simulink model "AAIR"  (R2020a)
settings: Solver=FixedStepAuto  StartTime=0.0  StopTime=60.0  FixedStep=1e-3  RelTol=1e-3  EnableMultiTasking=on
undefined symbols (not defined in the file): D0, D10, D11, D12, D13, D2, D4, D5, D6, D7, D8, D9, PTA0, PTA2, PTB23, PTB9, PTC16, PTC2, PTC3, PTC4, PTD0, PTD1, PTD2, PTD3
libraries: frdmk64flib x13, dspstat3 x1
settings Model: ExtModeTrigDuration=5  Creator=raymo  LastModifiedBy=raymo
settings OptimizationCC: EnhancedBackFolding=on  PassReuseOutputArgsAs=Individual arguments  ZeroExternalMemoryAtStartup=off  ZeroInternalMemoryAtStartup=off  MaxStackSize=64  OptimizeBlockOrder=speed  DifferentSizesBufferReuse=on  OptimizationCustomize=off  EfficientTunableParamExpr=on
settings DebuggingCC: ParameterTunabilityLossMsg=error
settings HardwareCC: ProdBitPerPointer=32  ProdBitPerSizeT=32  ProdBitPerPtrDiffT=32  ProdLargestAtomicInteger=Long  ProdLargestAtomicFloat=Double  ProdWordSize=32  ProdHWDeviceType=ARM Compatible->ARM Cortex
settings SFSimCC: MATLABDynamicMemAlloc=off
settings RTWCC: SystemTargetFile=ert.tlc  HardwareBoard=NXP FRDM-K64F  TemplateMakefile=ert_default_tmf  Toolchain=GNU Tools for ARM Embedded Processors
settings CodeAppCC: ForceParamTrailComments=on  IgnoreCustomStorageClasses=off  OperatorAnnotations=on  SimulinkDataObjDesc=on  SFDataObjDesc=on  InsertBlockDesc=on

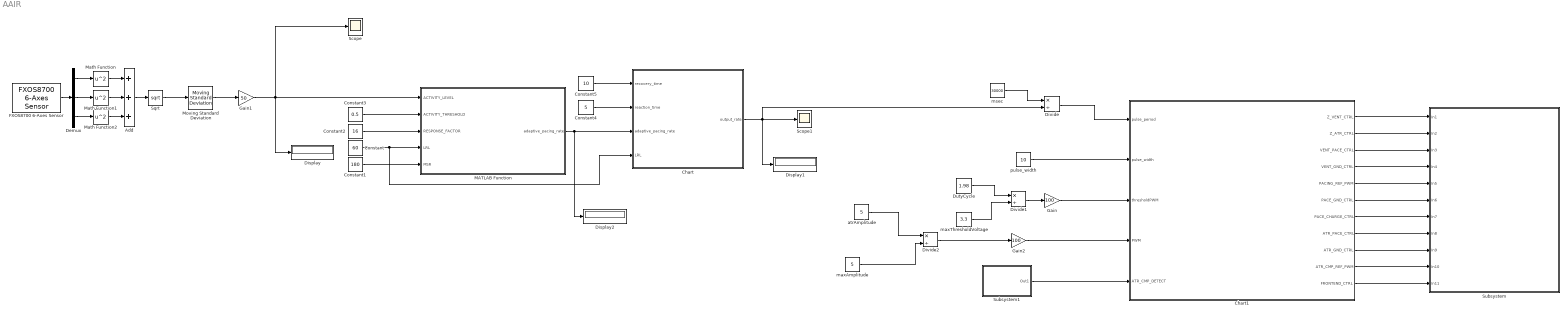
== system AAIR ==
  Add : Sum  Inputs=+++
  Chart : Stateflow chart  TreatAsAtomicUnit=on
  Chart1 : Stateflow chart  TreatAsAtomicUnit=on
  Constant : Constant  Value=60
  Constant1 : Constant  Value=180
  Constant2 : Constant  Value=16
  Constant3 : Constant  Value=0.5
  Constant4 : Constant  Value=5
  Constant5 : Constant  Value=10
  Demux : Demux  Outputs=3
  Display : Display
  Display1 : Display
  Display2 : Display
  Divide : Product  Inputs=*/
  Divide1 : Product  Inputs=*/
  Divide2 : Product  Inputs=*/
  DutyCycle : Constant  Value=1.98
  FXOS8700 6-Axes Sensor : frdmk64flib/FXOS8700 6-Axes Sensor  Activesensor=Accelerometer only  ODR=800Hz  HybridODR=400Hz  Accelfullrange=-4g to +4g  SampleTime=-1
  Gain : Gain  Gain=100
  Gain1 : Gain  Gain=50
  Gain2 : Gain  Gain=100
  MATLAB Function : MATLAB Function  TreatAsAtomicUnit=on
  Math Function : Math  Operator=square  SaturateOnIntegerOverflow=on
  Math Function1 : Math  Operator=square  SaturateOnIntegerOverflow=on
  Math Function2 : Math  Operator=square  SaturateOnIntegerOverflow=on
  Moving Standard Deviation : dspstat3/Moving Standard Deviation  Method=Sliding window  ForgettingFactorPort=off  SpecifyWindowLength=on  WindowLength=4  ForgettingFactor=0.9  SimulateUsing=Code generation
      settings: SourceProductBaseCode=DS
  Scope : Scope
  Scope1 : Scope
  Sqrt : Sqrt  SaturateOnIntegerOverflow=on
  Subsystem : Subsystem
  Subsystem1 : Subsystem
  atrAmplitude : Constant  Value=5
  maxAmplitude : Constant  Value=5
  maxThresholdVoltage : Constant  Value=3.3
  msec : Constant  Value=30000
  pulse_width : Constant  Value=10
  wires:
  Math Function2/1 -> Add/3
  Demux/3 -> Math Function2/1
  Constant2/1 -> MATLAB Function/3(RESPONSE_FACTOR)
  Constant/1 -> Chart/4(LRL), MATLAB Function/4(LRL)
  MATLAB Function/1(adaptive_pacing_rate) -> Chart/3(adaptive_pacing_rate), Display2/1
  Demux/1 -> Math Function/1
  Demux/2 -> Math Function1/1
  Math Function/1 -> Add/1
  Constant5/1 -> Chart/1(recovery_time)
  Add/1 -> Sqrt/1
  Constant4/1 -> Chart/2(reaction_time)
  Math Function1/1 -> Add/2
  Constant1/1 -> MATLAB Function/5(MSR)
  Sqrt/1 -> Moving Standard Deviation/1
  Gain1/1 -> Scope/1, Display/1, MATLAB Function/1(ACTIVITY_LEVEL)
  Constant3/1 -> MATLAB Function/2(ACTIVITY_THRESHOLD)
  FXOS8700 6-Axes Sensor/1 -> Demux/1
  Moving Standard Deviation/1 -> Gain1/1
  DutyCycle/1 -> Divide1/1
  Subsystem1/1(Out1) -> Chart1/5(ATR_CMP_DETECT)
  Gain/1 -> Chart1/3(thresholdPWM)
  Divide2/1 -> Gain2/1
  maxAmplitude/1 -> Divide2/2
  Divide/1 -> Chart1/1(pulse_period)
  Chart1/11(FRONTEND_CTRL) -> Subsystem/11(In11)
  Chart1/10(ATR_CMP_REF_PWM) -> Subsystem/10(In10)
  Chart1/9(ATR_GND_CTRL) -> Subsystem/9(In9)
  Chart1/8(ATR_PACE_CTRL) -> Subsystem/8(In8)
  Divide1/1 -> Gain/1
  Chart1/5(PACING_REF_PWM) -> Subsystem/5(In5)
  Chart1/6(PACE_GND_CTRL) -> Subsystem/6(In6)
  Gain2/1 -> Chart1/4(PWM)
  Chart1/3(VENT_PACE_CTRL) -> Subsystem/3(In3)
  Chart/1(output_rate) -> Divide/2, Display1/1, Scope1/1
  Chart1/1(Z_VENT_CTRL) -> Subsystem/1(In1)
  maxThresholdVoltage/1 -> Divide1/2
  Chart1/2(Z_ATR_CTRL) -> Subsystem/2(In2)
  msec/1 -> Divide/1
  Chart1/4(VENT_GND_CTRL) -> Subsystem/4(In4)
  pulse_width/1 -> Chart1/2(pulse_width)
  Chart1/7(PACE_CHARGE_CTRL) -> Subsystem/7(In7)
  atrAmplitude/1 -> Divide2/1

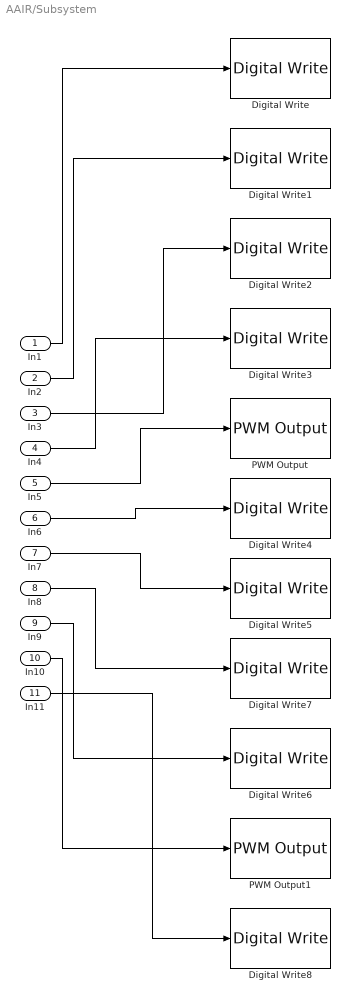
== system AAIR/Subsystem ==
  In1 : Inport
  In2 : Inport  Port=2
  In3 : Inport  Port=3
  In4 : Inport  Port=4
  In5 : Inport  Port=5
  In6 : Inport  Port=6
  In7 : Inport  Port=7
  In8 : Inport  Port=8
  In9 : Inport  Port=9
  In10 : Inport  Port=10
  In11 : Inport  Port=11
  Digital Write : frdmk64flib/Digital Write  Whichpin=PTC3 (D7)
  Digital Write1 : frdmk64flib/Digital Write  Whichpin=PTB23 (D4)
  Digital Write2 : frdmk64flib/Digital Write  Whichpin=PTC4 (D9)
  Digital Write3 : frdmk64flib/Digital Write  Whichpin=PTD3 (D12)
  Digital Write4 : frdmk64flib/Digital Write  Whichpin=PTD0 (D10)
  Digital Write5 : frdmk64flib/Digital Write  Whichpin=PTB9 (D2)
  Digital Write6 : frdmk64flib/Digital Write  Whichpin=PTD2 (D11)
  Digital Write7 : frdmk64flib/Digital Write  Whichpin=PTA0 (D8)
  Digital Write8 : frdmk64flib/Digital Write  Whichpin=PTD1 (D13)
  PWM Output : frdmk64flib/PWM Output  Whichpin=PTA2 (D5)  InitialFrequency=2000  InitialDutyCycle=50
  PWM Output1 : frdmk64flib/PWM Output  Whichpin=PTC2 (D6)  InitialFrequency=2000  InitialDutyCycle=50
  wires:
  In5/1 -> PWM Output/1
  In3/1 -> Digital Write2/1
  In1/1 -> Digital Write/1
  In4/1 -> Digital Write3/1
  In8/1 -> Digital Write7/1
  In9/1 -> Digital Write6/1
  In7/1 -> Digital Write5/1
  In2/1 -> Digital Write1/1
  In11/1 -> Digital Write8/1
  In10/1 -> PWM Output1/1
  In6/1 -> Digital Write4/1

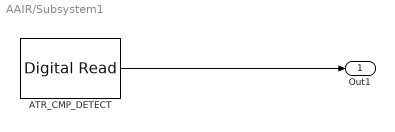
== system AAIR/Subsystem1 ==
  ATR_CMP_DETECT : frdmk64flib/Digital Read  Whichpin=PTC16 (D0)  SampleTime=-1
  Out1 : Outport
  wires:
  ATR_CMP_DETECT/1 -> Out1/1

== stateflow chart AAIR/Chart1 ==
  state Idle
    entry:
    %Set threshold
    ATR_CMP_REF_PWM = thresholdPWM;
    FRONTEND_CTRL = 1;
  state AVpacing
    entry:
    PACE_CHARGE_CTRL = 0;
    PACE_GND_CTRL = 1;
    ATR_PACE_CTRL = 1;
    ATR_GND_CTRL = 0;
    Z_ATR_CTRL = 0;
    Z_VENT_CTRL = 0;
    VENT_GND_CTRL = 0;
    VENT_PACE_CTRL = 0;
    PACING_REF_PWM = PWM;
  state ChargeDischarge
    entry:
    %C22
    ATR_PACE_CTRL = 0;
    VENT_PACE_CTRL = 0;
    PACING_REF_PWM = PWM;
    PACE_CHARGE_CTRL = 1;
    %C21
    PACE_GND_CTRL = 1;
    VENT_PACE_CTRL = 0;
    Z_ATR_CTRL = 0;
    Z_VENT_CTRL = 0;
    ATR_GND_CTRL = 1;
    VENT_GND_CTRL = 0;
  (default) -> Idle
  Idle -> ChargeDischarge
  ChargeDischarge -> ChargeDischarge [order 1] : after(5,msec)[ATR_CMP_DETECT == 1]
  ChargeDischarge -> AVpacing [order 2] : [after(pulse_period-pulse_width,msec)]
  AVpacing -> ChargeDischarge : [after(pulse_width, msec)]
  data: pulse_period input; pulse_width input; thresholdPWM input; PWM input; Z_VENT_CTRL output; Z_ATR_CTRL output; VENT_PACE_CTRL output; VENT_GND_CTRL output; PACING_REF_PWM output; PACE_GND_CTRL output; PACE_CHARGE_CTRL output; ATR_PACE_CTRL output; ATR_GND_CTRL output; ATR_CMP_REF_PWM output; ATR_CMP_DETECT input; FRONTEND_CTRL output

== matlab function AAIR/MATLAB Function ==
  data: ACTIVITY_LEVEL input; adaptive_pacing_rate output; ACTIVITY_THRESHOLD input; RESPONSE_FACTOR input; LRL input; MSR input
function adaptive_pacing_rate = fcn(ACTIVITY_LEVEL, ACTIVITY_THRESHOLD, RESPONSE_FACTOR, LRL , MSR)
    if ACTIVITY_LEVEL <= ACTIVITY_THRESHOLD
        adaptive_pacing_rate = LRL; 
    else
        slope = 2.5*RESPONSE_FACTOR;
        b = LRL - (slope*ACTIVITY_THRESHOLD);
        linear_rate_response = (slope*ACTIVITY_LEVEL) + b;
        if(linear_rate_response >= MSR)
           adaptive_pacing_rate = MSR;
        else
            adaptive_pacing_rate = linear_rate_response;
        end
    end
end

== stateflow chart AAIR/Chart ==
  state IDLE
    entry:
    output_rate = LRL;
  state INIT
    entry:
    %The slope of the time response curves
    step_up = abs((adaptive_pacing_rate - output_rate)/reaction_time);
    step_down = abs((adaptive_pacing_rate - output_rate)/recovery_time);
  state STEP_DOWN
    entry:
    output_rate = output_rate - step_down;
  state STEP_UP
    entry:
    output_rate = output_rate + step_up;
  (default) -> IDLE
  IDLE -> INIT
  INIT -> STEP_UP [order 1] : [output_rate < adaptive_pacing_rate]
  INIT -> STEP_DOWN [order 2] : [output_rate > adaptive_pacing_rate]
  STEP_UP -> INIT : [after(1000,msec)]
  STEP_DOWN -> INIT : [after(1000,msec)]
  data: output_rate output; recovery_time input; reaction_time input; adaptive_pacing_rate input; LRL input; step_up local; step_down local
